simulink model "w2p3"  (R2020b)
settings: Solver=ode45  StartTime=0.0  StopTime=120  RelTol=1e-3
undefined symbols (not defined in the file or in its folder): b, m
settings Model: Creator=WELCOME  LastModifiedBy=WELCOME

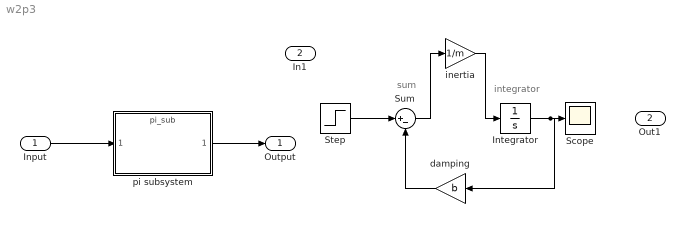
== system w2p3 ==
  note: integrator
  note: sum
  Input : Inport
  In1 : Inport  Port=2
  Integrator : Integrator
  Scope : Scope
  Step : Step  Time=0  SampleTime=0
  Sum : Sum  Inputs=|+-
  damping : Gain  Gain=b
  inertia : Gain  Gain=1/m
  pi subsystem : ModelReference  ModelNameDialog=pi_sub  SimulationMode=Normal  ModelReferenceVersion=1.3
  Output : Outport
  Out1 : Outport  Port=2
  wires:
  Input/1 -> pi subsystem/1
  pi subsystem/1 -> Output/1
  Sum/1 -> inertia/1
  inertia/1 -> Integrator/1
  damping/1 -> Sum/2
  Integrator/1 -> Scope/1, damping/1
  Step/1 -> Sum/1
